simulink model "linearisierterRegelkreis"  (R2014b)
settings: Solver=ode45  StartTime=0.0  StopTime=100  RelTol=1e-3
libraries: cstblocks x2
settings Model: Creator=hollowman  LastModifiedBy=sigurd

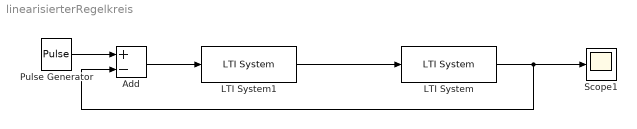
== system linearisierterRegelkreis ==
  Add : Sum  Inputs=+-
  LTI System : cstblocks/LTI System  sys=G  IC=[]
  LTI System1 : cstblocks/LTI System  sys=C  IC=[]
  Pulse Generator : DiscretePulseGenerator  PulseType=Time based  Amplitude=0.001  Period=10  PulseWidth=50
  Scope1 : Scope
  wires:
  LTI System1/1 -> LTI System/1
  LTI System/1 -> Add/2, Scope1/1
  Pulse Generator/1 -> Add/1
  Add/1 -> LTI System1/1
